simulink model "hcc_sm_v6_circuit"  (R2024b)
settings: Solver=VariableStepAuto  StartTime=0.0  StopTime=1  RelTol=1e-3
libraries: spsSeriesRLCBranchLib x530, spsGtoLib x144, spsNonlinearResistorLib x78, spsGroundLib x2, spsDCVoltageSourceLib x1, spsThreePhaseTransformerTwoWindingsLib x1, spsThreePhaseSourceLib x1, spspowerguiLib x1
(part 1 of 3)
settings Model: Creator=56305  LastModifiedBy=XixiLab
settings OptimizationCC: ReuseModelBlockBuffer=off
settings RTWCC: GPUComputeCapability=3.5

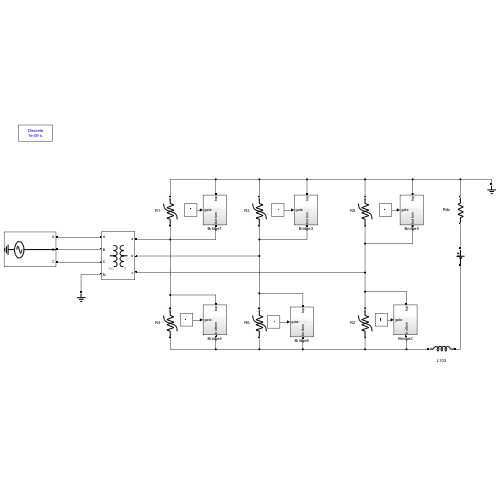
[thumbnail: Simulink's stored preview of the top-level diagram]
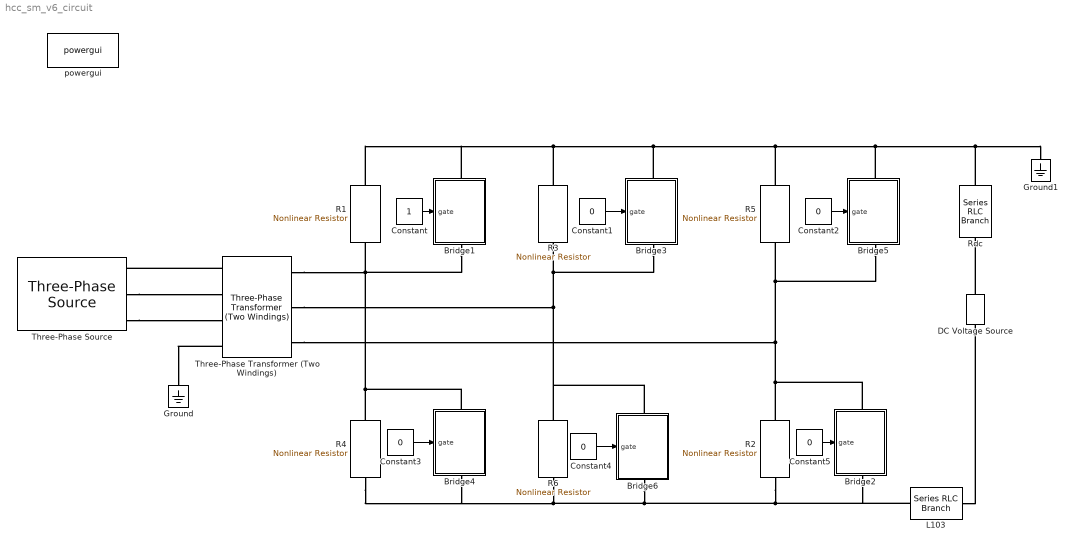
== system hcc_sm_v6_circuit ==
  Bridge1 : Subsystem
      settings: PortSchema="{\"entries\":[{\"content\":{\"sides\":[{\"content\":{\"connectorIds\":[\"In1\"]},\"type\":\"ConnectorPlacement.EquallySpacedRectSide\",\"uuid\":\"41aa3e2a-70f0-4b77-aa16-68e99ec54bcf\"},{\"content\":{\"side\":\"RIGHT\"},\"type\":\"ConnectorPlacement.EquallySpacedRectSide\",\"uuid\":\"96eb3ac2-20ab-4313-b955-709dae12ba5a\"},{\"content\":{\"connectorIds\":[\"LConn1\"],\"side\":\"TOP\"},\"type\":\"ConnectorPlacement.EquallySpacedRectSide\",\"uuid\":\"75cf1ed1-d1d6-43fb-a0f7-eae0627f950f\"},{\"content\":{\"connectorIds\":[\"RConn1\"],\"side\":\"BOTTOM\"},\"type\":\"ConnectorPlacement.EquallySpacedRectSide\",\"uuid\":\"e3d24c16-695e-4958-a9e5-c1041aebacaf\"}]},\"type\":\"ConnectorPlacement.EquallySpacedConnector\",\"uuid\":\"cea135f8-b684-4f22-bc6f-773380cf8880\"}],\"packageUris\":[\"http://schema.mathworks.com/mf0/Connector/R2020b\"],\"version\":\"1.0\"}"
  Bridge2 : Subsystem
      settings: PortSchema="{\"entries\":[{\"content\":{\"sides\":[{\"content\":{\"connectorIds\":[\"In1\"]},\"type\":\"ConnectorPlacement.EquallySpacedRectSide\",\"uuid\":\"41aa3e2a-70f0-4b77-aa16-68e99ec54bcf\"},{\"content\":{\"side\":\"RIGHT\"},\"type\":\"ConnectorPlacement.EquallySpacedRectSide\",\"uuid\":\"96eb3ac2-20ab-4313-b955-709dae12ba5a\"},{\"content\":{\"connectorIds\":[\"LConn1\"],\"side\":\"TOP\"},\"type\":\"ConnectorPlacement.EquallySpacedRectSide\",\"uuid\":\"75cf1ed1-d1d6-43fb-a0f7-eae0627f950f\"},{\"content\":{\"connectorIds\":[\"RConn1\"],\"side\":\"BOTTOM\"},\"type\":\"ConnectorPlacement.EquallySpacedRectSide\",\"uuid\":\"e3d24c16-695e-4958-a9e5-c1041aebacaf\"}]},\"type\":\"ConnectorPlacement.EquallySpacedConnector\",\"uuid\":\"cea135f8-b684-4f22-bc6f-773380cf8880\"}],\"packageUris\":[\"http://schema.mathworks.com/mf0/Connector/R2020b\"],\"version\":\"1.0\"}"
  Bridge3 : Subsystem
      settings: PortSchema="{\"entries\":[{\"content\":{\"sides\":[{\"content\":{\"connectorIds\":[\"In1\"]},\"type\":\"ConnectorPlacement.EquallySpacedRectSide\",\"uuid\":\"41aa3e2a-70f0-4b77-aa16-68e99ec54bcf\"},{\"content\":{\"side\":\"RIGHT\"},\"type\":\"ConnectorPlacement.EquallySpacedRectSide\",\"uuid\":\"96eb3ac2-20ab-4313-b955-709dae12ba5a\"},{\"content\":{\"connectorIds\":[\"LConn1\"],\"side\":\"TOP\"},\"type\":\"ConnectorPlacement.EquallySpacedRectSide\",\"uuid\":\"75cf1ed1-d1d6-43fb-a0f7-eae0627f950f\"},{\"content\":{\"connectorIds\":[\"RConn1\"],\"side\":\"BOTTOM\"},\"type\":\"ConnectorPlacement.EquallySpacedRectSide\",\"uuid\":\"e3d24c16-695e-4958-a9e5-c1041aebacaf\"}]},\"type\":\"ConnectorPlacement.EquallySpacedConnector\",\"uuid\":\"cea135f8-b684-4f22-bc6f-773380cf8880\"}],\"packageUris\":[\"http://schema.mathworks.com/mf0/Connector/R2020b\"],\"version\":\"1.0\"}"
  Bridge4 : Subsystem
      settings: PortSchema="{\"entries\":[{\"content\":{\"sides\":[{\"content\":{\"connectorIds\":[\"In1\"]},\"type\":\"ConnectorPlacement.EquallySpacedRectSide\",\"uuid\":\"41aa3e2a-70f0-4b77-aa16-68e99ec54bcf\"},{\"content\":{\"side\":\"RIGHT\"},\"type\":\"ConnectorPlacement.EquallySpacedRectSide\",\"uuid\":\"96eb3ac2-20ab-4313-b955-709dae12ba5a\"},{\"content\":{\"connectorIds\":[\"LConn1\"],\"side\":\"TOP\"},\"type\":\"ConnectorPlacement.EquallySpacedRectSide\",\"uuid\":\"75cf1ed1-d1d6-43fb-a0f7-eae0627f950f\"},{\"content\":{\"connectorIds\":[\"RConn1\"],\"side\":\"BOTTOM\"},\"type\":\"ConnectorPlacement.EquallySpacedRectSide\",\"uuid\":\"e3d24c16-695e-4958-a9e5-c1041aebacaf\"}]},\"type\":\"ConnectorPlacement.EquallySpacedConnector\",\"uuid\":\"cea135f8-b684-4f22-bc6f-773380cf8880\"}],\"packageUris\":[\"http://schema.mathworks.com/mf0/Connector/R2020b\"],\"version\":\"1.0\"}"
  Bridge5 : Subsystem
      settings: PortSchema="{\"entries\":[{\"content\":{\"sides\":[{\"content\":{\"connectorIds\":[\"In1\"]},\"type\":\"ConnectorPlacement.EquallySpacedRectSide\",\"uuid\":\"41aa3e2a-70f0-4b77-aa16-68e99ec54bcf\"},{\"content\":{\"side\":\"RIGHT\"},\"type\":\"ConnectorPlacement.EquallySpacedRectSide\",\"uuid\":\"96eb3ac2-20ab-4313-b955-709dae12ba5a\"},{\"content\":{\"connectorIds\":[\"LConn1\"],\"side\":\"TOP\"},\"type\":\"ConnectorPlacement.EquallySpacedRectSide\",\"uuid\":\"75cf1ed1-d1d6-43fb-a0f7-eae0627f950f\"},{\"content\":{\"connectorIds\":[\"RConn1\"],\"side\":\"BOTTOM\"},\"type\":\"ConnectorPlacement.EquallySpacedRectSide\",\"uuid\":\"e3d24c16-695e-4958-a9e5-c1041aebacaf\"}]},\"type\":\"ConnectorPlacement.EquallySpacedConnector\",\"uuid\":\"cea135f8-b684-4f22-bc6f-773380cf8880\"}],\"packageUris\":[\"http://schema.mathworks.com/mf0/Connector/R2020b\"],\"version\":\"1.0\"}"
  Bridge6 : Subsystem
      settings: PortSchema="{\"entries\":[{\"content\":{\"sides\":[{\"content\":{\"connectorIds\":[\"In1\"]},\"type\":\"ConnectorPlacement.EquallySpacedRectSide\",\"uuid\":\"41aa3e2a-70f0-4b77-aa16-68e99ec54bcf\"},{\"content\":{\"side\":\"RIGHT\"},\"type\":\"ConnectorPlacement.EquallySpacedRectSide\",\"uuid\":\"96eb3ac2-20ab-4313-b955-709dae12ba5a\"},{\"content\":{\"connectorIds\":[\"LConn1\"],\"side\":\"TOP\"},\"type\":\"ConnectorPlacement.EquallySpacedRectSide\",\"uuid\":\"75cf1ed1-d1d6-43fb-a0f7-eae0627f950f\"},{\"content\":{\"connectorIds\":[\"RConn1\"],\"side\":\"BOTTOM\"},\"type\":\"ConnectorPlacement.EquallySpacedRectSide\",\"uuid\":\"e3d24c16-695e-4958-a9e5-c1041aebacaf\"}]},\"type\":\"ConnectorPlacement.EquallySpacedConnector\",\"uuid\":\"cea135f8-b684-4f22-bc6f-773380cf8880\"}],\"packageUris\":[\"http://schema.mathworks.com/mf0/Connector/R2020b\"],\"version\":\"1.0\"}"
  Constant : Constant
  Constant{1..5} (5 alike) : Constant  Value=0
  DC Voltage Source : spsDCVoltageSourceLib/DC Voltage Source  Amplitude=5700  Measurements=None
  Ground : spsGroundLib/Ground  LConnTagsString=a
  Ground1 : spsGroundLib/Ground  LConnTagsString=a
  L103 : spsSeriesRLCBranchLib/Series RLC Branch  LConnTagsString=__new0  RConnTagsString=__new0  BranchType=L  Resistance=36  Inductance=120e-03  SetiL0=off  InitialCurrent=0  Capacitance=2.62e-06  Setx0=off  InitialVoltage=0  Measurements=None
  R{1..6} (6 alike) : spsNonlinearResistorLib/Nonlinear Resistor  SrcType=Current source  VI=[9800 0.001;11564 200;12299 1000;13259.4098 4000.01;13259.4196 4000.02;13259.4294 4000.03;13259.4392 4000.04;13259.449 4000.05;13259.4588 4000.06;13259.4686 4000.07;13259.4784 4000.08]
      settings: LibrarySourceBlock=sps_lib/Passives/Nonlinear Resistor
  Rdc : spsSeriesRLCBranchLib/Series RLC Branch  LConnTagsString=__new0  RConnTagsString=__new0  BranchType=R  Resistance=1  Inductance=120e-03  SetiL0=off  InitialCurrent=0  Capacitance=2.62e-06  Setx0=off  InitialVoltage=0  Measurements=None
  Three-Phase Transformer (Two Windings) : spsThreePhaseTransformerTwoWindingsLib/Three-Phase Transformer (Two Windings)  Winding1Connection=Yn  Winding2Connection=Y  CoreType=Three single-phase transformers  SetSaturation=off  Hysteresis=off  DataFile='hysteresis'  SetInitialFlux=off  Measurements=None  UNITS=pu  NominalPower=[ 215.4e6 , 50 ]  Winding1=[ 345e3 , 0.002 , 0.08 ]  Winding2=[ 50.8e3 , 0.002 , 0.08 ]  Rm=500  Lm=500  L0=0.5  Saturation=[ 0,0 ; 0.0024,1.2 ; 1.0,1.52 ]  InitialFluxes=[ 0.8 , -0.8 , 0.7 ]  BreakLoop=off  DiscreteSolver=Trapezoidal iterative  DataType=off  TransfoNumber=1
  Three-Phase Source : spsThreePhaseSourceLib/Three-Phase Source  InternalConnection=Yg  VoltagePhases=off  Voltage=345e3  PhaseAngle=0  Voltage_phases=[25e3 25e3 25e3]/sqrt(3)  PhaseAngles_phases=[0 -120 +120]  Frequency=50  NonIdealSource=off  SpecifyImpedance=off  Resistance=0  Inductance=0  ShortCircuitLevel=100e6  BaseVoltage=25e3  XRratio=7  BusType=swing  Pref=10e3  Qref=0  Prefabc=[10e3, 10e3, 10e3]  Qrefabc=[0, 0, 0]  Qmin=-inf  Qmax=inf
  powergui : spspowerguiLib/powergui  Priority=1  SimulationMode=Discrete  SampleTime=1e-9  frequency=60  Iterations=50  frequencyindice=0  Pbase=100e6  ErrMax=1e-4  UnitsV=kV  UnitsW=MW  buscounter=0  FunctionMessages=off  echomessages=off  EnableUseOfTLC=off  CurrentSourceSwitches=off  DisableSnubberDevices=off  DisableRonSwitches=off  DisableVfSwitches=off  DisplayEquations=off  AutomaticDiscreteSolvers=off  SolverType=Tustin/Backward Euler (TBE)  Interpol=off  ExternalGateDelay=off  methode=off  Ts=100  x0status=blocks  SPID=on  SwTol=0  HookPort=off  NonlinearTolerance=1e-4  nMaxIteration=100  ContinueOnMaxIteration=off  RestoreLinks=warning  ResistiveCurrentMeasurement=off  Frange=[0:2:500]  Ylog=off  Xlog=on  ShowGrid=off  save=off  variable=ZData  structure=0  ZoomFFT=off  StartTime=0.0  cycles=1  DisplayStyle=1  fundamental=60  FreqAxis=off  MaxFrequency=1000  frequencyindicesteady=1  RmsSteady=1  display=off
  wires:
  Constant/1 -> Bridge1/1(gate)
  Constant1/1 -> Bridge3/1(gate)
  Constant2/1 -> Bridge5/1(gate)
  Constant3/1 -> Bridge4/1(gate)
  Constant4/1 -> Bridge6/1(gate)
  Constant5/1 -> Bridge2/1(gate)
  connections:
  Three-Phase Transformer (Two Windings)/LConn1 -- Three-Phase Source/RConn1
  Three-Phase Source/RConn2 -- Three-Phase Transformer (Two Windings)/LConn2
  Three-Phase Source/RConn3 -- Three-Phase Transformer (Two Windings)/LConn3
  Three-Phase Transformer (Two Windings)/LConn4 -- Ground/LConn1
  R4/LConn1 -- Bridge4/LConn1 -- Bridge1/RConn1 -- R1/RConn1 -- Three-Phase Transformer (Two Windings)/RConn1
  Three-Phase Transformer (Two Windings)/RConn2 -- Bridge6/LConn1 -- R6/LConn1 -- Bridge3/RConn1 -- R3/RConn1
  R2/LConn1 -- Bridge2/LConn1 -- Three-Phase Transformer (Two Windings)/RConn3 -- Bridge5/RConn1 -- R5/RConn1
  R2/RConn1 -- Bridge2/RConn1 -- L103/LConn1 -- Bridge6/RConn1 -- Bridge4/RConn1 -- R4/RConn1 -- R6/RConn1
  DC Voltage Source/RConn1 -- Rdc/RConn1
  R3/LConn1 -- R1/LConn1 -- Bridge1/LConn1 -- Bridge3/LConn1 -- R5/LConn1 -- Bridge5/LConn1 -- Rdc/LConn1 -- Ground1/LConn1
  L103/RConn1 -- DC Voltage Source/LConn1

== system hcc_sm_v6_circuit/Bridge1 ==
  gate : Inport
  Segment1 : Subsystem
  Segment2 : Subsystem
  Segment3 : Subsystem
  Segment4 : Subsystem
  top : PMIOPort  Side=Left
  bottom : PMIOPort  Port=2  Side=Right
  wires:
  gate/1 -> Segment2/1(gate), Segment4/1(gate), Segment3/1(gate), Segment1/1(gate)
  connections:
  Segment2/LConn1 -- Segment1/RConn1
  Segment3/LConn1 -- Segment2/RConn1
  Segment4/LConn1 -- Segment3/RConn1
  top/RConn1 -- Segment1/LConn1
  Segment4/RConn1 -- bottom/RConn1

== system hcc_sm_v6_circuit/Bridge2 ==
  gate : Inport
  Segment1 : Subsystem
  Segment2 : Subsystem
  Segment3 : Subsystem
  Segment4 : Subsystem
  top : PMIOPort  Side=Left
  bottom : PMIOPort  Port=2  Side=Right
  wires:
  gate/1 -> Segment2/1(gate), Segment4/1(gate), Segment3/1(gate), Segment1/1(gate)
  connections:
  Segment2/LConn1 -- Segment1/RConn1
  Segment3/LConn1 -- Segment2/RConn1
  Segment4/LConn1 -- Segment3/RConn1
  top/RConn1 -- Segment1/LConn1
  Segment4/RConn1 -- bottom/RConn1

== system hcc_sm_v6_circuit/Bridge3 ==
  gate : Inport
  Segment1 : Subsystem
  Segment2 : Subsystem
  Segment3 : Subsystem
  Segment4 : Subsystem
  top : PMIOPort  Side=Left
  bottom : PMIOPort  Port=2  Side=Right
  wires:
  gate/1 -> Segment2/1(gate), Segment4/1(gate), Segment3/1(gate), Segment1/1(gate)
  connections:
  Segment2/LConn1 -- Segment1/RConn1
  Segment3/LConn1 -- Segment2/RConn1
  Segment4/LConn1 -- Segment3/RConn1
  top/RConn1 -- Segment1/LConn1
  Segment4/RConn1 -- bottom/RConn1

== system hcc_sm_v6_circuit/Bridge4 ==
  gate : Inport
  Segment1 : Subsystem
  Segment2 : Subsystem
  Segment3 : Subsystem
  Segment4 : Subsystem
  top : PMIOPort  Side=Left
  bottom : PMIOPort  Port=2  Side=Right
  wires:
  gate/1 -> Segment2/1(gate), Segment4/1(gate), Segment3/1(gate), Segment1/1(gate)
  connections:
  Segment2/LConn1 -- Segment1/RConn1
  Segment3/LConn1 -- Segment2/RConn1
  Segment4/LConn1 -- Segment3/RConn1
  top/RConn1 -- Segment1/LConn1
  Segment4/RConn1 -- bottom/RConn1

== system hcc_sm_v6_circuit/Bridge5 ==
  gate : Inport
  Segment1 : Subsystem
  Segment2 : Subsystem
  Segment3 : Subsystem
  Segment4 : Subsystem
  top : PMIOPort  Side=Left
  bottom : PMIOPort  Port=2  Side=Right
  wires:
  gate/1 -> Segment2/1(gate), Segment4/1(gate), Segment3/1(gate), Segment1/1(gate)
  connections:
  Segment2/LConn1 -- Segment1/RConn1
  Segment3/LConn1 -- Segment2/RConn1
  Segment4/LConn1 -- Segment3/RConn1
  top/RConn1 -- Segment1/LConn1
  Segment4/RConn1 -- bottom/RConn1

== system hcc_sm_v6_circuit/Bridge6 ==
  gate : Inport
  Segment1 : Subsystem
  Segment2 : Subsystem
  Segment3 : Subsystem
  Segment4 : Subsystem
  top : PMIOPort  Side=Left
  bottom : PMIOPort  Port=2  Side=Right
  wires:
  gate/1 -> Segment2/1(gate), Segment4/1(gate), Segment3/1(gate), Segment1/1(gate)
  connections:
  Segment2/LConn1 -- Segment1/RConn1
  Segment3/LConn1 -- Segment2/RConn1
  Segment4/LConn1 -- Segment3/RConn1
  top/RConn1 -- Segment1/LConn1
  Segment4/RConn1 -- bottom/RConn1

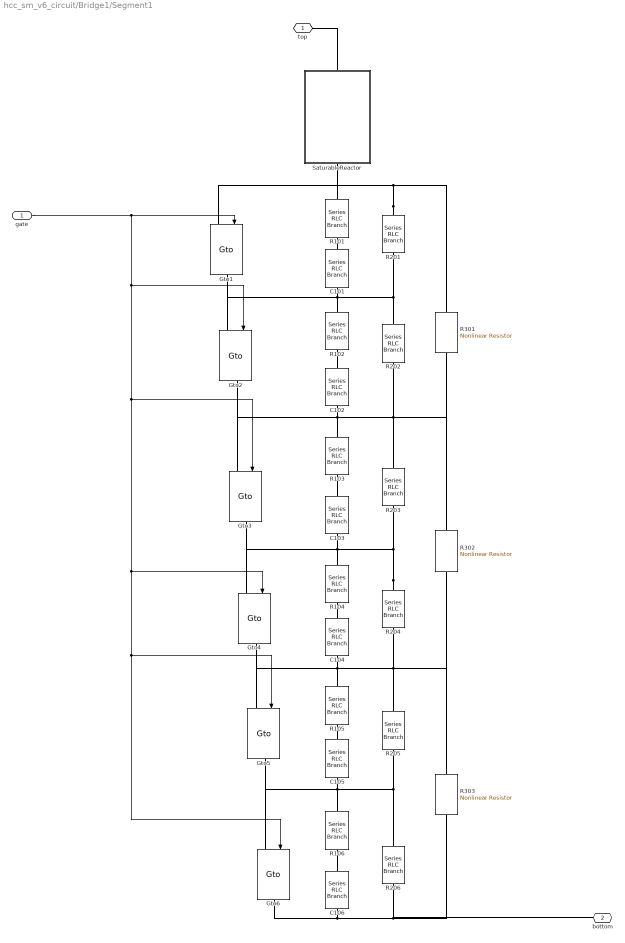
== system hcc_sm_v6_circuit/Bridge1/Segment1 ==
  gate : Inport
  C{101..106} (6 alike) : spsSeriesRLCBranchLib/Series RLC Branch  LConnTagsString=__new0  RConnTagsString=__new0  BranchType=C  Resistance=350  Inductance=107.42e-03  SetiL0=off  InitialCurrent=0  Capacitance=2.2*1e-6  Setx0=off  InitialVoltage=0  Measurements=None
  Gto{1..6} (6 alike) : spsGtoLib/Gto  Ron=0.226e-6  Lon=0  Vf=1.2  Tf=10e-6  Tt=20e-6  IC=0  Rs=161.25e3  Cs=0  Measurements=off
      settings: LibrarySourceBlock=sps_lib/Power Electronics/Gto
  R{101..106} (6 alike) : spsSeriesRLCBranchLib/Series RLC Branch  LConnTagsString=__new0  RConnTagsString=__new0  BranchType=R  Resistance=36  Inductance=107.42e-03  SetiL0=off  InitialCurrent=0  Capacitance=2.62e-06  Setx0=off  InitialVoltage=0  Measurements=None
  R{201..206} (6 alike) : spsSeriesRLCBranchLib/Series RLC Branch  LConnTagsString=__new0  RConnTagsString=__new0  BranchType=R  Resistance=88  Inductance=107.42e-03  SetiL0=off  InitialCurrent=0  Capacitance=2.62e-06  Setx0=off  InitialVoltage=0  Measurements=None
  R301 : spsNonlinearResistorLib/Nonlinear Resistor  SrcType=Current source  VI=[4400 0.001;5199.92 10;5449.84 100;5700.2 250;5849.8 500;5925.04 750;5999.84 1000;6199.64 2000;6274.84 2500;6325 3000;6600 5500]
      settings: LibrarySourceBlock=sps_lib/Passives/Nonlinear Resistor
  R302 : spsNonlinearResistorLib/Nonlinear Resistor  SrcType=Current source  VI=[4400 0.001;5199.92 10;5449.84 100;5700.2 250;5849.8 500;5925.04 750;5999.84 1000;6199.64 2000;6274.84 2500;6325 3000;6600 5500]
      settings: LibrarySourceBlock=sps_lib/Passives/Nonlinear Resistor
  R303 : spsNonlinearResistorLib/Nonlinear Resistor  SrcType=Current source  VI=[4400 0.001;5199.92 10;5449.84 100;5700.2 250;5849.8 500;5925.04 750;5999.84 1000;6199.64 2000;6274.84 2500;6325 3000;6600 5500]
      settings: LibrarySourceBlock=sps_lib/Passives/Nonlinear Resistor
  SaturableReactor : Subsystem
  top : PMIOPort  Side=Left
  bottom : PMIOPort  Port=2  Side=Right
  wires:
  gate/1 -> Gto3/1, Gto4/1, Gto6/1, Gto5/1, Gto2/1, Gto1/1
  connections:
  R201/RConn1 -- Gto2/LConn1 -- Gto1/RConn1 -- C101/RConn1 -- R102/LConn1 -- R202/LConn1
  R204/LConn1 -- R203/RConn1 -- C103/RConn1 -- Gto4/LConn1 -- Gto3/RConn1 -- R104/LConn1
  R201/LConn1 -- R301/LConn1 -- Gto1/LConn1 -- SaturableReactor/RConn1 -- R101/LConn1
  R205/RConn1 -- C105/RConn1 -- R106/LConn1 -- Gto6/LConn1 -- Gto5/RConn1 -- R206/LConn1
  R202/RConn1 -- R203/LConn1 -- R302/LConn1 -- R301/RConn1 -- C102/RConn1 -- Gto3/LConn1 -- Gto2/RConn1 -- R103/LConn1
  R105/LConn1 -- C104/RConn1 -- Gto5/LConn1 -- Gto4/RConn1 -- R205/LConn1 -- R303/LConn1 -- R302/RConn1 -- R204/RConn1
  R303/RConn1 -- bottom/RConn1 -- R206/RConn1 -- C106/RConn1 -- Gto6/RConn1
  SaturableReactor/LConn1 -- top/RConn1
  C101/LConn1 -- R101/RConn1
  C102/LConn1 -- R102/RConn1
  R103/RConn1 -- C103/LConn1
  R104/RConn1 -- C104/LConn1
  R105/RConn1 -- C105/LConn1
  R106/RConn1 -- C106/LConn1

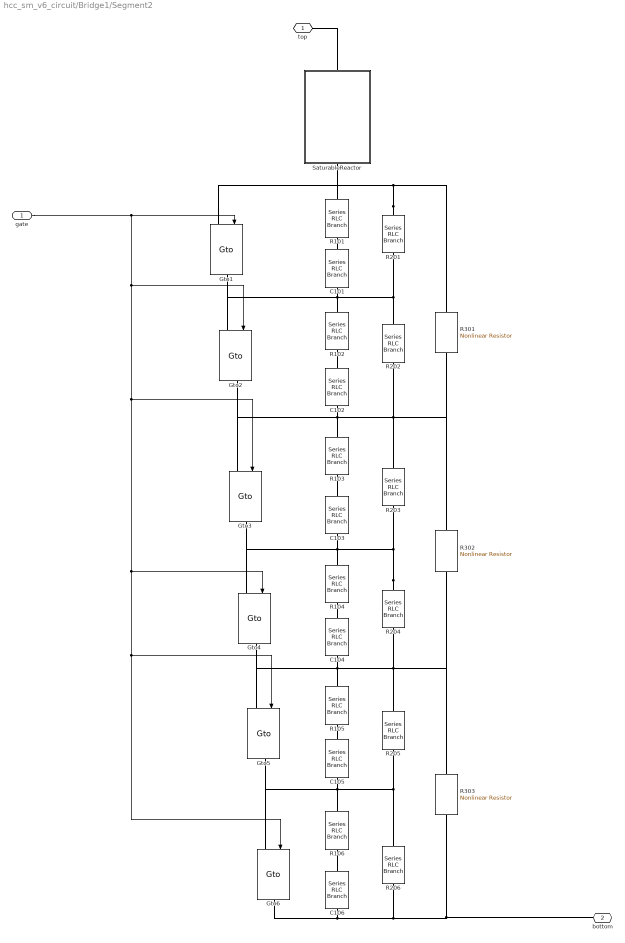
== system hcc_sm_v6_circuit/Bridge1/Segment2 ==
  gate : Inport
  C{101..106} (6 alike) : spsSeriesRLCBranchLib/Series RLC Branch  LConnTagsString=__new0  RConnTagsString=__new0  BranchType=C  Resistance=350  Inductance=107.42e-03  SetiL0=off  InitialCurrent=0  Capacitance=2.2*1e-6  Setx0=off  InitialVoltage=0  Measurements=None
  Gto{1..6} (6 alike) : spsGtoLib/Gto  Ron=0.226e-6  Lon=0  Vf=1.2  Tf=10e-6  Tt=20e-6  IC=0  Rs=161.25e3  Cs=0  Measurements=off
  R{101..106} (6 alike) : spsSeriesRLCBranchLib/Series RLC Branch  LConnTagsString=__new0  RConnTagsString=__new0  BranchType=R  Resistance=36  Inductance=107.42e-03  SetiL0=off  InitialCurrent=0  Capacitance=2.62e-06  Setx0=off  InitialVoltage=0  Measurements=None
  R{201..206} (6 alike) : spsSeriesRLCBranchLib/Series RLC Branch  LConnTagsString=__new0  RConnTagsString=__new0  BranchType=R  Resistance=88  Inductance=107.42e-03  SetiL0=off  InitialCurrent=0  Capacitance=2.62e-06  Setx0=off  InitialVoltage=0  Measurements=None
  R301 : spsNonlinearResistorLib/Nonlinear Resistor  SrcType=Current source  VI=[4400 0.001;5199.92 10;5449.84 100;5700.2 250;5849.8 500;5925.04 750;5999.84 1000;6199.64 2000;6274.84 2500;6325 3000;6600 5500]
  R302 : spsNonlinearResistorLib/Nonlinear Resistor  SrcType=Current source  VI=[4400 0.001;5199.92 10;5449.84 100;5700.2 250;5849.8 500;5925.04 750;5999.84 1000;6199.64 2000;6274.84 2500;6325 3000;6600 5500]
  R303 : spsNonlinearResistorLib/Nonlinear Resistor  SrcType=Current source  VI=[4400 0.001;5199.92 10;5449.84 100;5700.2 250;5849.8 500;5925.04 750;5999.84 1000;6199.64 2000;6274.84 2500;6325 3000;6600 5500]
  SaturableReactor : Subsystem
  top : PMIOPort  Side=Left
  bottom : PMIOPort  Port=2  Side=Right
  wires:
  gate/1 -> Gto3/1, Gto4/1, Gto6/1, Gto5/1, Gto2/1, Gto1/1
  connections:
  R201/RConn1 -- Gto2/LConn1 -- Gto1/RConn1 -- C101/RConn1 -- R102/LConn1 -- R202/LConn1
  R204/LConn1 -- R203/RConn1 -- C103/RConn1 -- Gto4/LConn1 -- Gto3/RConn1 -- R104/LConn1
  R201/LConn1 -- R301/LConn1 -- Gto1/LConn1 -- SaturableReactor/RConn1 -- R101/LConn1
  R205/RConn1 -- C105/RConn1 -- R106/LConn1 -- Gto6/LConn1 -- Gto5/RConn1 -- R206/LConn1
  R202/RConn1 -- R203/LConn1 -- R302/LConn1 -- R301/RConn1 -- C102/RConn1 -- Gto3/LConn1 -- Gto2/RConn1 -- R103/LConn1
  R105/LConn1 -- C104/RConn1 -- Gto5/LConn1 -- Gto4/RConn1 -- R205/LConn1 -- R303/LConn1 -- R302/RConn1 -- R204/RConn1
  R303/RConn1 -- bottom/RConn1 -- R206/RConn1 -- C106/RConn1 -- Gto6/RConn1
  SaturableReactor/LConn1 -- top/RConn1
  C101/LConn1 -- R101/RConn1
  C102/LConn1 -- R102/RConn1
  R103/RConn1 -- C103/LConn1
  R104/RConn1 -- C104/LConn1
  R105/RConn1 -- C105/LConn1
  R106/RConn1 -- C106/LConn1

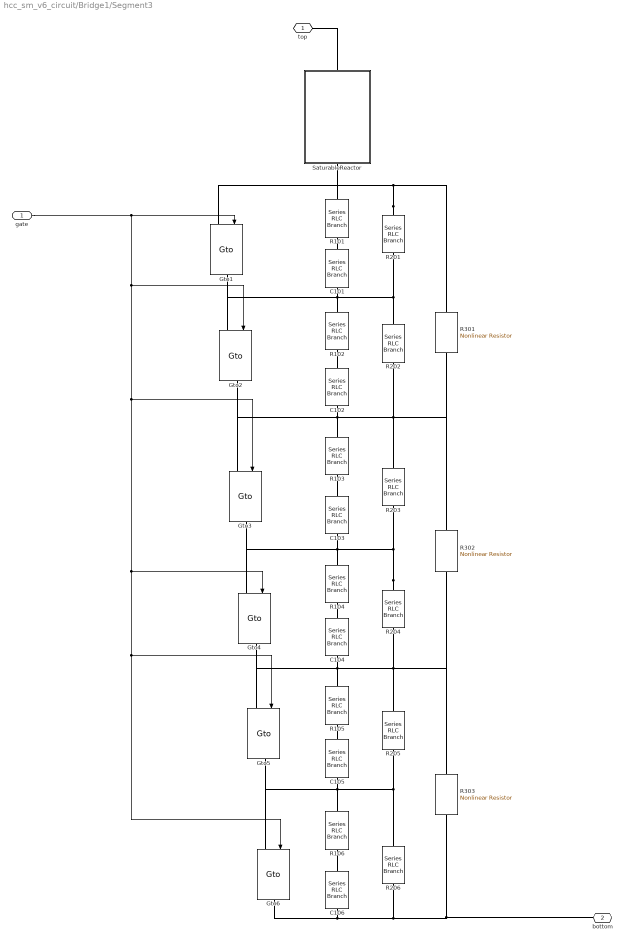
== system hcc_sm_v6_circuit/Bridge1/Segment3 ==
  gate : Inport
  C{101..106} (6 alike) : spsSeriesRLCBranchLib/Series RLC Branch  LConnTagsString=__new0  RConnTagsString=__new0  BranchType=C  Resistance=350  Inductance=107.42e-03  SetiL0=off  InitialCurrent=0  Capacitance=2.2*1e-6  Setx0=off  InitialVoltage=0  Measurements=None
  Gto{1..6} (6 alike) : spsGtoLib/Gto  Ron=0.226e-6  Lon=0  Vf=1.2  Tf=10e-6  Tt=20e-6  IC=0  Rs=161.25e3  Cs=0  Measurements=off
  R{101..106} (6 alike) : spsSeriesRLCBranchLib/Series RLC Branch  LConnTagsString=__new0  RConnTagsString=__new0  BranchType=R  Resistance=36  Inductance=107.42e-03  SetiL0=off  InitialCurrent=0  Capacitance=2.62e-06  Setx0=off  InitialVoltage=0  Measurements=None
  R{201..206} (6 alike) : spsSeriesRLCBranchLib/Series RLC Branch  LConnTagsString=__new0  RConnTagsString=__new0  BranchType=R  Resistance=88  Inductance=107.42e-03  SetiL0=off  InitialCurrent=0  Capacitance=2.62e-06  Setx0=off  InitialVoltage=0  Measurements=None
  R301 : spsNonlinearResistorLib/Nonlinear Resistor  SrcType=Current source  VI=[4400 0.001;5199.92 10;5449.84 100;5700.2 250;5849.8 500;5925.04 750;5999.84 1000;6199.64 2000;6274.84 2500;6325 3000;6600 5500]
  R302 : spsNonlinearResistorLib/Nonlinear Resistor  SrcType=Current source  VI=[4400 0.001;5199.92 10;5449.84 100;5700.2 250;5849.8 500;5925.04 750;5999.84 1000;6199.64 2000;6274.84 2500;6325 3000;6600 5500]
  R303 : spsNonlinearResistorLib/Nonlinear Resistor  SrcType=Current source  VI=[4400 0.001;5199.92 10;5449.84 100;5700.2 250;5849.8 500;5925.04 750;5999.84 1000;6199.64 2000;6274.84 2500;6325 3000;6600 5500]
  SaturableReactor : Subsystem
  top : PMIOPort  Side=Left
  bottom : PMIOPort  Port=2  Side=Right
  wires:
  gate/1 -> Gto3/1, Gto4/1, Gto6/1, Gto5/1, Gto2/1, Gto1/1
  connections:
  R201/RConn1 -- Gto2/LConn1 -- Gto1/RConn1 -- C101/RConn1 -- R102/LConn1 -- R202/LConn1
  R204/LConn1 -- R203/RConn1 -- C103/RConn1 -- Gto4/LConn1 -- Gto3/RConn1 -- R104/LConn1
  R201/LConn1 -- R301/LConn1 -- Gto1/LConn1 -- SaturableReactor/RConn1 -- R101/LConn1
  R205/RConn1 -- C105/RConn1 -- R106/LConn1 -- Gto6/LConn1 -- Gto5/RConn1 -- R206/LConn1
  R202/RConn1 -- R203/LConn1 -- R302/LConn1 -- R301/RConn1 -- C102/RConn1 -- Gto3/LConn1 -- Gto2/RConn1 -- R103/LConn1
  R105/LConn1 -- C104/RConn1 -- Gto5/LConn1 -- Gto4/RConn1 -- R205/LConn1 -- R303/LConn1 -- R302/RConn1 -- R204/RConn1
  R303/RConn1 -- bottom/RConn1 -- R206/RConn1 -- C106/RConn1 -- Gto6/RConn1
  SaturableReactor/LConn1 -- top/RConn1
  C101/LConn1 -- R101/RConn1
  C102/LConn1 -- R102/RConn1
  R103/RConn1 -- C103/LConn1
  R104/RConn1 -- C104/LConn1
  R105/RConn1 -- C105/LConn1
  R106/RConn1 -- C106/LConn1

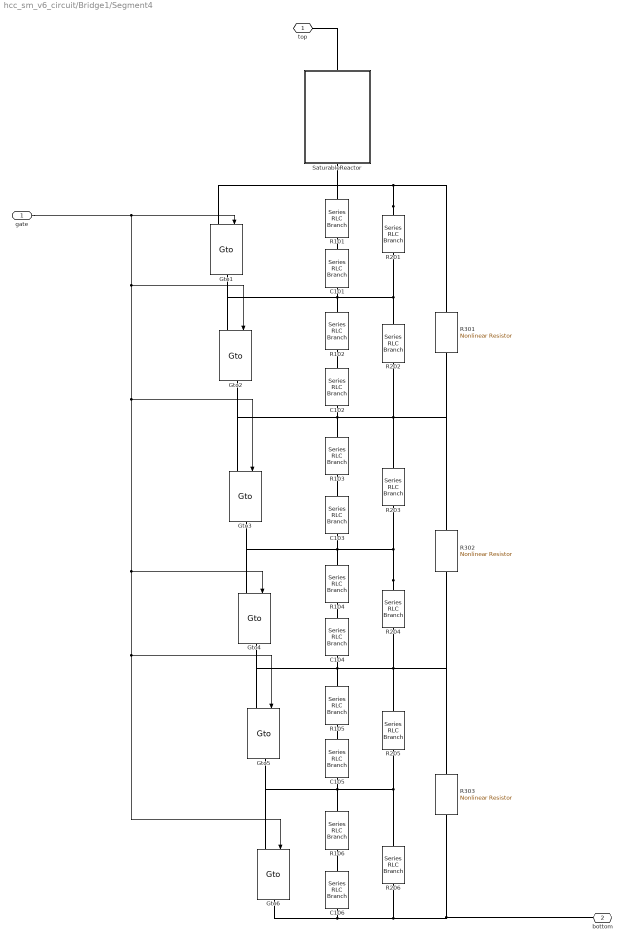
== system hcc_sm_v6_circuit/Bridge1/Segment4 ==
  gate : Inport
  C{101..106} (6 alike) : spsSeriesRLCBranchLib/Series RLC Branch  LConnTagsString=__new0  RConnTagsString=__new0  BranchType=C  Resistance=350  Inductance=107.42e-03  SetiL0=off  InitialCurrent=0  Capacitance=2.2*1e-6  Setx0=off  InitialVoltage=0  Measurements=None
  Gto{1..6} (6 alike) : spsGtoLib/Gto  Ron=0.226e-6  Lon=0  Vf=1.2  Tf=10e-6  Tt=20e-6  IC=0  Rs=161.25e3  Cs=0  Measurements=off
  R{101..106} (6 alike) : spsSeriesRLCBranchLib/Series RLC Branch  LConnTagsString=__new0  RConnTagsString=__new0  BranchType=R  Resistance=36  Inductance=107.42e-03  SetiL0=off  InitialCurrent=0  Capacitance=2.62e-06  Setx0=off  InitialVoltage=0  Measurements=None
  R{201..206} (6 alike) : spsSeriesRLCBranchLib/Series RLC Branch  LConnTagsString=__new0  RConnTagsString=__new0  BranchType=R  Resistance=88  Inductance=107.42e-03  SetiL0=off  InitialCurrent=0  Capacitance=2.62e-06  Setx0=off  InitialVoltage=0  Measurements=None
  R301 : spsNonlinearResistorLib/Nonlinear Resistor  SrcType=Current source  VI=[4400 0.001;5199.92 10;5449.84 100;5700.2 250;5849.8 500;5925.04 750;5999.84 1000;6199.64 2000;6274.84 2500;6325 3000;6600 5500]
  R302 : spsNonlinearResistorLib/Nonlinear Resistor  SrcType=Current source  VI=[4400 0.001;5199.92 10;5449.84 100;5700.2 250;5849.8 500;5925.04 750;5999.84 1000;6199.64 2000;6274.84 2500;6325 3000;6600 5500]
  R303 : spsNonlinearResistorLib/Nonlinear Resistor  SrcType=Current source  VI=[4400 0.001;5199.92 10;5449.84 100;5700.2 250;5849.8 500;5925.04 750;5999.84 1000;6199.64 2000;6274.84 2500;6325 3000;6600 5500]
  SaturableReactor : Subsystem
  top : PMIOPort  Side=Left
  bottom : PMIOPort  Port=2  Side=Right
  wires:
  gate/1 -> Gto3/1, Gto4/1, Gto6/1, Gto5/1, Gto2/1, Gto1/1
  connections:
  R201/RConn1 -- Gto2/LConn1 -- Gto1/RConn1 -- C101/RConn1 -- R102/LConn1 -- R202/LConn1
  R204/LConn1 -- R203/RConn1 -- C103/RConn1 -- Gto4/LConn1 -- Gto3/RConn1 -- R104/LConn1
  R201/LConn1 -- R301/LConn1 -- Gto1/LConn1 -- SaturableReactor/RConn1 -- R101/LConn1
  R205/RConn1 -- C105/RConn1 -- R106/LConn1 -- Gto6/LConn1 -- Gto5/RConn1 -- R206/LConn1
  R202/RConn1 -- R203/LConn1 -- R302/LConn1 -- R301/RConn1 -- C102/RConn1 -- Gto3/LConn1 -- Gto2/RConn1 -- R103/LConn1
  R105/LConn1 -- C104/RConn1 -- Gto5/LConn1 -- Gto4/RConn1 -- R205/LConn1 -- R303/LConn1 -- R302/RConn1 -- R204/RConn1
  R303/RConn1 -- bottom/RConn1 -- R206/RConn1 -- C106/RConn1 -- Gto6/RConn1
  SaturableReactor/LConn1 -- top/RConn1
  C101/LConn1 -- R101/RConn1
  C102/LConn1 -- R102/RConn1
  R103/RConn1 -- C103/LConn1
  R104/RConn1 -- C104/LConn1
  R105/RConn1 -- C105/LConn1
  R106/RConn1 -- C106/LConn1

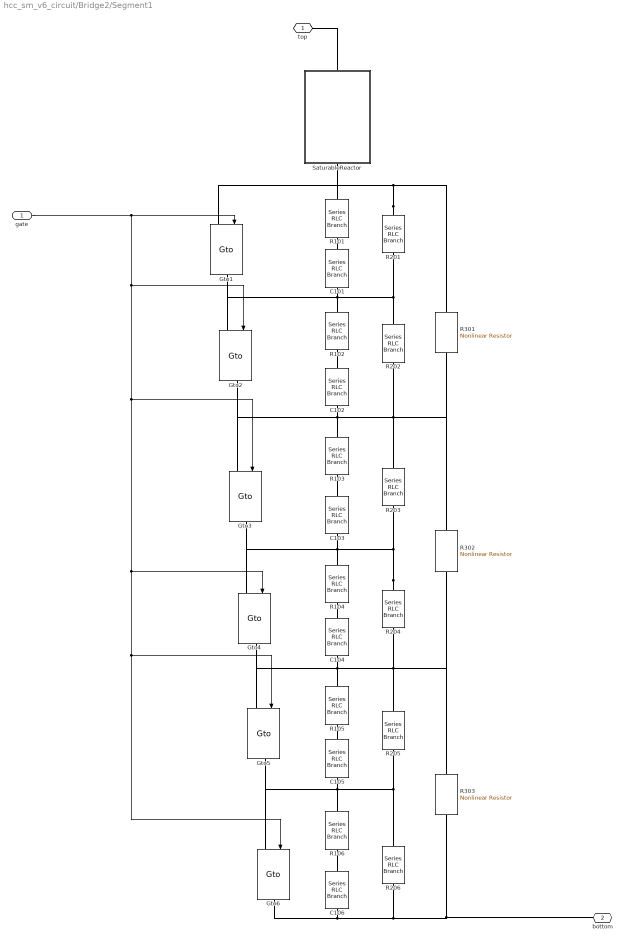
== system hcc_sm_v6_circuit/Bridge2/Segment1 ==
  gate : Inport
  C{101..106} (6 alike) : spsSeriesRLCBranchLib/Series RLC Branch  LConnTagsString=__new0  RConnTagsString=__new0  BranchType=C  Resistance=350  Inductance=107.42e-03  SetiL0=off  InitialCurrent=0  Capacitance=2.2*1e-6  Setx0=off  InitialVoltage=0  Measurements=None
  Gto{1..6} (6 alike) : spsGtoLib/Gto  Ron=0.226e-6  Lon=0  Vf=1.2  Tf=10e-6  Tt=20e-6  IC=0  Rs=161.25e3  Cs=0  Measurements=off
  R{101..106} (6 alike) : spsSeriesRLCBranchLib/Series RLC Branch  LConnTagsString=__new0  RConnTagsString=__new0  BranchType=R  Resistance=36  Inductance=107.42e-03  SetiL0=off  InitialCurrent=0  Capacitance=2.62e-06  Setx0=off  InitialVoltage=0  Measurements=None
  R{201..206} (6 alike) : spsSeriesRLCBranchLib/Series RLC Branch  LConnTagsString=__new0  RConnTagsString=__new0  BranchType=R  Resistance=88  Inductance=107.42e-03  SetiL0=off  InitialCurrent=0  Capacitance=2.62e-06  Setx0=off  InitialVoltage=0  Measurements=None
  R301 : spsNonlinearResistorLib/Nonlinear Resistor  SrcType=Current source  VI=[4400 0.001;5199.92 10;5449.84 100;5700.2 250;5849.8 500;5925.04 750;5999.84 1000;6199.64 2000;6274.84 2500;6325 3000;6600 5500]
  R302 : spsNonlinearResistorLib/Nonlinear Resistor  SrcType=Current source  VI=[4400 0.001;5199.92 10;5449.84 100;5700.2 250;5849.8 500;5925.04 750;5999.84 1000;6199.64 2000;6274.84 2500;6325 3000;6600 5500]
  R303 : spsNonlinearResistorLib/Nonlinear Resistor  SrcType=Current source  VI=[4400 0.001;5199.92 10;5449.84 100;5700.2 250;5849.8 500;5925.04 750;5999.84 1000;6199.64 2000;6274.84 2500;6325 3000;6600 5500]
  SaturableReactor : Subsystem
  top : PMIOPort  Side=Left
  bottom : PMIOPort  Port=2  Side=Right
  wires:
  gate/1 -> Gto3/1, Gto4/1, Gto6/1, Gto5/1, Gto2/1, Gto1/1
  connections:
  R201/RConn1 -- Gto2/LConn1 -- Gto1/RConn1 -- C101/RConn1 -- R102/LConn1 -- R202/LConn1
  R204/LConn1 -- R203/RConn1 -- C103/RConn1 -- Gto4/LConn1 -- Gto3/RConn1 -- R104/LConn1
  R201/LConn1 -- R301/LConn1 -- Gto1/LConn1 -- SaturableReactor/RConn1 -- R101/LConn1
  R205/RConn1 -- C105/RConn1 -- R106/LConn1 -- Gto6/LConn1 -- Gto5/RConn1 -- R206/LConn1
  R202/RConn1 -- R203/LConn1 -- R302/LConn1 -- R301/RConn1 -- C102/RConn1 -- Gto3/LConn1 -- Gto2/RConn1 -- R103/LConn1
  R105/LConn1 -- C104/RConn1 -- Gto5/LConn1 -- Gto4/RConn1 -- R205/LConn1 -- R303/LConn1 -- R302/RConn1 -- R204/RConn1
  R303/RConn1 -- bottom/RConn1 -- R206/RConn1 -- C106/RConn1 -- Gto6/RConn1
  SaturableReactor/LConn1 -- top/RConn1
  C101/LConn1 -- R101/RConn1
  C102/LConn1 -- R102/RConn1
  R103/RConn1 -- C103/LConn1
  R104/RConn1 -- C104/LConn1
  R105/RConn1 -- C105/LConn1
  R106/RConn1 -- C106/LConn1

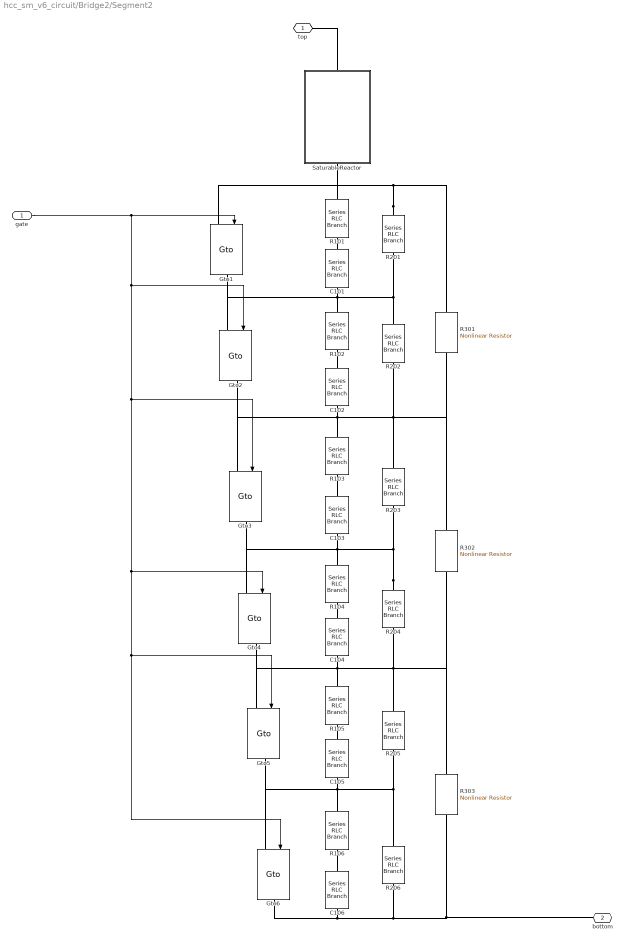
== system hcc_sm_v6_circuit/Bridge2/Segment2 ==
  gate : Inport
  C{101..106} (6 alike) : spsSeriesRLCBranchLib/Series RLC Branch  LConnTagsString=__new0  RConnTagsString=__new0  BranchType=C  Resistance=350  Inductance=107.42e-03  SetiL0=off  InitialCurrent=0  Capacitance=2.2*1e-6  Setx0=off  InitialVoltage=0  Measurements=None
  Gto{1..6} (6 alike) : spsGtoLib/Gto  Ron=0.226e-6  Lon=0  Vf=1.2  Tf=10e-6  Tt=20e-6  IC=0  Rs=161.25e3  Cs=0  Measurements=off
  R{101..106} (6 alike) : spsSeriesRLCBranchLib/Series RLC Branch  LConnTagsString=__new0  RConnTagsString=__new0  BranchType=R  Resistance=36  Inductance=107.42e-03  SetiL0=off  InitialCurrent=0  Capacitance=2.62e-06  Setx0=off  InitialVoltage=0  Measurements=None
  R{201..206} (6 alike) : spsSeriesRLCBranchLib/Series RLC Branch  LConnTagsString=__new0  RConnTagsString=__new0  BranchType=R  Resistance=88  Inductance=107.42e-03  SetiL0=off  InitialCurrent=0  Capacitance=2.62e-06  Setx0=off  InitialVoltage=0  Measurements=None
  R301 : spsNonlinearResistorLib/Nonlinear Resistor  SrcType=Current source  VI=[4400 0.001;5199.92 10;5449.84 100;5700.2 250;5849.8 500;5925.04 750;5999.84 1000;6199.64 2000;6274.84 2500;6325 3000;6600 5500]
  R302 : spsNonlinearResistorLib/Nonlinear Resistor  SrcType=Current source  VI=[4400 0.001;5199.92 10;5449.84 100;5700.2 250;5849.8 500;5925.04 750;5999.84 1000;6199.64 2000;6274.84 2500;6325 3000;6600 5500]
  R303 : spsNonlinearResistorLib/Nonlinear Resistor  SrcType=Current source  VI=[4400 0.001;5199.92 10;5449.84 100;5700.2 250;5849.8 500;5925.04 750;5999.84 1000;6199.64 2000;6274.84 2500;6325 3000;6600 5500]
  SaturableReactor : Subsystem
  top : PMIOPort  Side=Left
  bottom : PMIOPort  Port=2  Side=Right
  wires:
  gate/1 -> Gto3/1, Gto4/1, Gto6/1, Gto5/1, Gto2/1, Gto1/1
  connections:
  R201/RConn1 -- Gto2/LConn1 -- Gto1/RConn1 -- C101/RConn1 -- R102/LConn1 -- R202/LConn1
  R204/LConn1 -- R203/RConn1 -- C103/RConn1 -- Gto4/LConn1 -- Gto3/RConn1 -- R104/LConn1
  R201/LConn1 -- R301/LConn1 -- Gto1/LConn1 -- SaturableReactor/RConn1 -- R101/LConn1
  R205/RConn1 -- C105/RConn1 -- R106/LConn1 -- Gto6/LConn1 -- Gto5/RConn1 -- R206/LConn1
  R202/RConn1 -- R203/LConn1 -- R302/LConn1 -- R301/RConn1 -- C102/RConn1 -- Gto3/LConn1 -- Gto2/RConn1 -- R103/LConn1
  R105/LConn1 -- C104/RConn1 -- Gto5/LConn1 -- Gto4/RConn1 -- R205/LConn1 -- R303/LConn1 -- R302/RConn1 -- R204/RConn1
  R303/RConn1 -- bottom/RConn1 -- R206/RConn1 -- C106/RConn1 -- Gto6/RConn1
  SaturableReactor/LConn1 -- top/RConn1
  C101/LConn1 -- R101/RConn1
  C102/LConn1 -- R102/RConn1
  R103/RConn1 -- C103/LConn1
  R104/RConn1 -- C104/LConn1
  R105/RConn1 -- C105/LConn1
  R106/RConn1 -- C106/LConn1

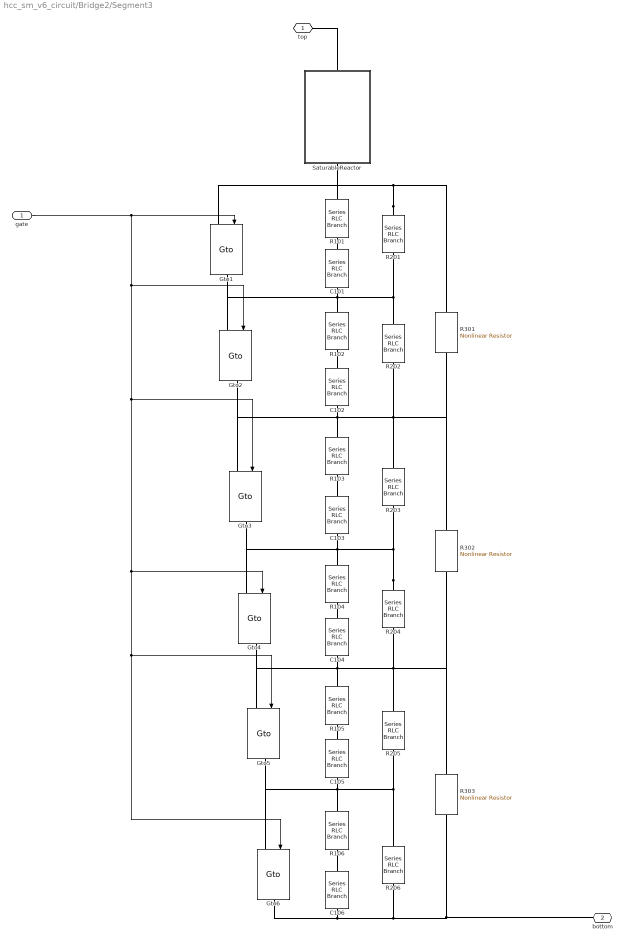
== system hcc_sm_v6_circuit/Bridge2/Segment3 ==
  gate : Inport
  C{101..106} (6 alike) : spsSeriesRLCBranchLib/Series RLC Branch  LConnTagsString=__new0  RConnTagsString=__new0  BranchType=C  Resistance=350  Inductance=107.42e-03  SetiL0=off  InitialCurrent=0  Capacitance=2.2*1e-6  Setx0=off  InitialVoltage=0  Measurements=None
  Gto{1..6} (6 alike) : spsGtoLib/Gto  Ron=0.226e-6  Lon=0  Vf=1.2  Tf=10e-6  Tt=20e-6  IC=0  Rs=161.25e3  Cs=0  Measurements=off
  R{101..106} (6 alike) : spsSeriesRLCBranchLib/Series RLC Branch  LConnTagsString=__new0  RConnTagsString=__new0  BranchType=R  Resistance=36  Inductance=107.42e-03  SetiL0=off  InitialCurrent=0  Capacitance=2.62e-06  Setx0=off  InitialVoltage=0  Measurements=None
  R{201..206} (6 alike) : spsSeriesRLCBranchLib/Series RLC Branch  LConnTagsString=__new0  RConnTagsString=__new0  BranchType=R  Resistance=88  Inductance=107.42e-03  SetiL0=off  InitialCurrent=0  Capacitance=2.62e-06  Setx0=off  InitialVoltage=0  Measurements=None
  R301 : spsNonlinearResistorLib/Nonlinear Resistor  SrcType=Current source  VI=[4400 0.001;5199.92 10;5449.84 100;5700.2 250;5849.8 500;5925.04 750;5999.84 1000;6199.64 2000;6274.84 2500;6325 3000;6600 5500]
  R302 : spsNonlinearResistorLib/Nonlinear Resistor  SrcType=Current source  VI=[4400 0.001;5199.92 10;5449.84 100;5700.2 250;5849.8 500;5925.04 750;5999.84 1000;6199.64 2000;6274.84 2500;6325 3000;6600 5500]
  R303 : spsNonlinearResistorLib/Nonlinear Resistor  SrcType=Current source  VI=[4400 0.001;5199.92 10;5449.84 100;5700.2 250;5849.8 500;5925.04 750;5999.84 1000;6199.64 2000;6274.84 2500;6325 3000;6600 5500]
  SaturableReactor : Subsystem
  top : PMIOPort  Side=Left
  bottom : PMIOPort  Port=2  Side=Right
  wires:
  gate/1 -> Gto3/1, Gto4/1, Gto6/1, Gto5/1, Gto2/1, Gto1/1
  connections:
  R201/RConn1 -- Gto2/LConn1 -- Gto1/RConn1 -- C101/RConn1 -- R102/LConn1 -- R202/LConn1
  R204/LConn1 -- R203/RConn1 -- C103/RConn1 -- Gto4/LConn1 -- Gto3/RConn1 -- R104/LConn1
  R201/LConn1 -- R301/LConn1 -- Gto1/LConn1 -- SaturableReactor/RConn1 -- R101/LConn1
  R205/RConn1 -- C105/RConn1 -- R106/LConn1 -- Gto6/LConn1 -- Gto5/RConn1 -- R206/LConn1
  R202/RConn1 -- R203/LConn1 -- R302/LConn1 -- R301/RConn1 -- C102/RConn1 -- Gto3/LConn1 -- Gto2/RConn1 -- R103/LConn1
  R105/LConn1 -- C104/RConn1 -- Gto5/LConn1 -- Gto4/RConn1 -- R205/LConn1 -- R303/LConn1 -- R302/RConn1 -- R204/RConn1
  R303/RConn1 -- bottom/RConn1 -- R206/RConn1 -- C106/RConn1 -- Gto6/RConn1
  SaturableReactor/LConn1 -- top/RConn1
  C101/LConn1 -- R101/RConn1
  C102/LConn1 -- R102/RConn1
  R103/RConn1 -- C103/LConn1
  R104/RConn1 -- C104/LConn1
  R105/RConn1 -- C105/LConn1
  R106/RConn1 -- C106/LConn1

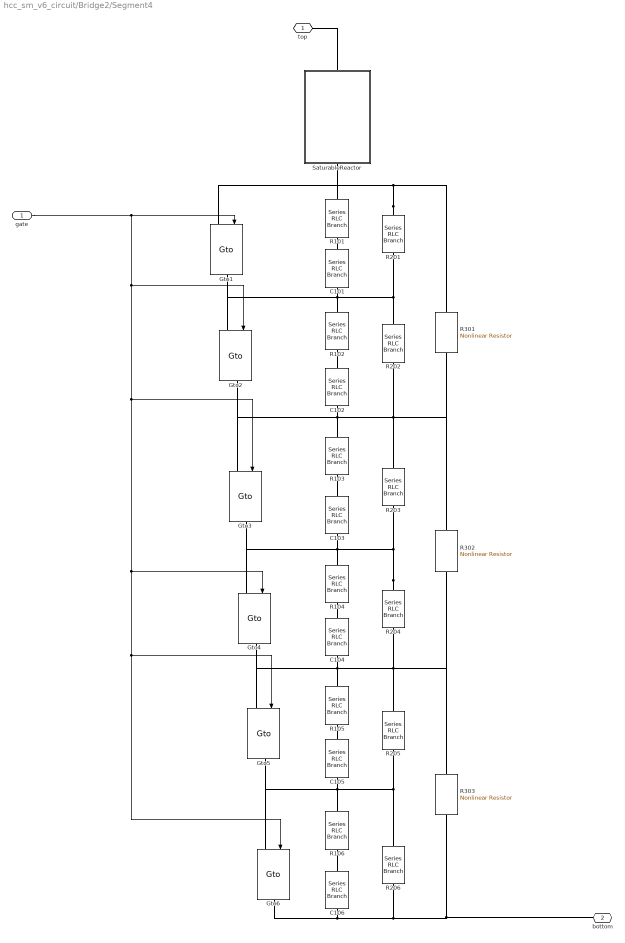
== system hcc_sm_v6_circuit/Bridge2/Segment4 ==
  gate : Inport
  C{101..106} (6 alike) : spsSeriesRLCBranchLib/Series RLC Branch  LConnTagsString=__new0  RConnTagsString=__new0  BranchType=C  Resistance=350  Inductance=107.42e-03  SetiL0=off  InitialCurrent=0  Capacitance=2.2*1e-6  Setx0=off  InitialVoltage=0  Measurements=None
  Gto{1..6} (6 alike) : spsGtoLib/Gto  Ron=0.226e-6  Lon=0  Vf=1.2  Tf=10e-6  Tt=20e-6  IC=0  Rs=161.25e3  Cs=0  Measurements=off
  R{101..106} (6 alike) : spsSeriesRLCBranchLib/Series RLC Branch  LConnTagsString=__new0  RConnTagsString=__new0  BranchType=R  Resistance=36  Inductance=107.42e-03  SetiL0=off  InitialCurrent=0  Capacitance=2.62e-06  Setx0=off  InitialVoltage=0  Measurements=None
  R{201..206} (6 alike) : spsSeriesRLCBranchLib/Series RLC Branch  LConnTagsString=__new0  RConnTagsString=__new0  BranchType=R  Resistance=88  Inductance=107.42e-03  SetiL0=off  InitialCurrent=0  Capacitance=2.62e-06  Setx0=off  InitialVoltage=0  Measurements=None
  R301 : spsNonlinearResistorLib/Nonlinear Resistor  SrcType=Current source  VI=[4400 0.001;5199.92 10;5449.84 100;5700.2 250;5849.8 500;5925.04 750;5999.84 1000;6199.64 2000;6274.84 2500;6325 3000;6600 5500]
  R302 : spsNonlinearResistorLib/Nonlinear Resistor  SrcType=Current source  VI=[4400 0.001;5199.92 10;5449.84 100;5700.2 250;5849.8 500;5925.04 750;5999.84 1000;6199.64 2000;6274.84 2500;6325 3000;6600 5500]
  R303 : spsNonlinearResistorLib/Nonlinear Resistor  SrcType=Current source  VI=[4400 0.001;5199.92 10;5449.84 100;5700.2 250;5849.8 500;5925.04 750;5999.84 1000;6199.64 2000;6274.84 2500;6325 3000;6600 5500]
  SaturableReactor : Subsystem
  top : PMIOPort  Side=Left
  bottom : PMIOPort  Port=2  Side=Right
  wires:
  gate/1 -> Gto3/1, Gto4/1, Gto6/1, Gto5/1, Gto2/1, Gto1/1
  connections:
  R201/RConn1 -- Gto2/LConn1 -- Gto1/RConn1 -- C101/RConn1 -- R102/LConn1 -- R202/LConn1
  R204/LConn1 -- R203/RConn1 -- C103/RConn1 -- Gto4/LConn1 -- Gto3/RConn1 -- R104/LConn1
  R201/LConn1 -- R301/LConn1 -- Gto1/LConn1 -- SaturableReactor/RConn1 -- R101/LConn1
  R205/RConn1 -- C105/RConn1 -- R106/LConn1 -- Gto6/LConn1 -- Gto5/RConn1 -- R206/LConn1
  R202/RConn1 -- R203/LConn1 -- R302/LConn1 -- R301/RConn1 -- C102/RConn1 -- Gto3/LConn1 -- Gto2/RConn1 -- R103/LConn1
  R105/LConn1 -- C104/RConn1 -- Gto5/LConn1 -- Gto4/RConn1 -- R205/LConn1 -- R303/LConn1 -- R302/RConn1 -- R204/RConn1
  R303/RConn1 -- bottom/RConn1 -- R206/RConn1 -- C106/RConn1 -- Gto6/RConn1
  SaturableReactor/LConn1 -- top/RConn1
  C101/LConn1 -- R101/RConn1
  C102/LConn1 -- R102/RConn1
  R103/RConn1 -- C103/LConn1
  R104/RConn1 -- C104/LConn1
  R105/RConn1 -- C105/LConn1
  R106/RConn1 -- C106/LConn1

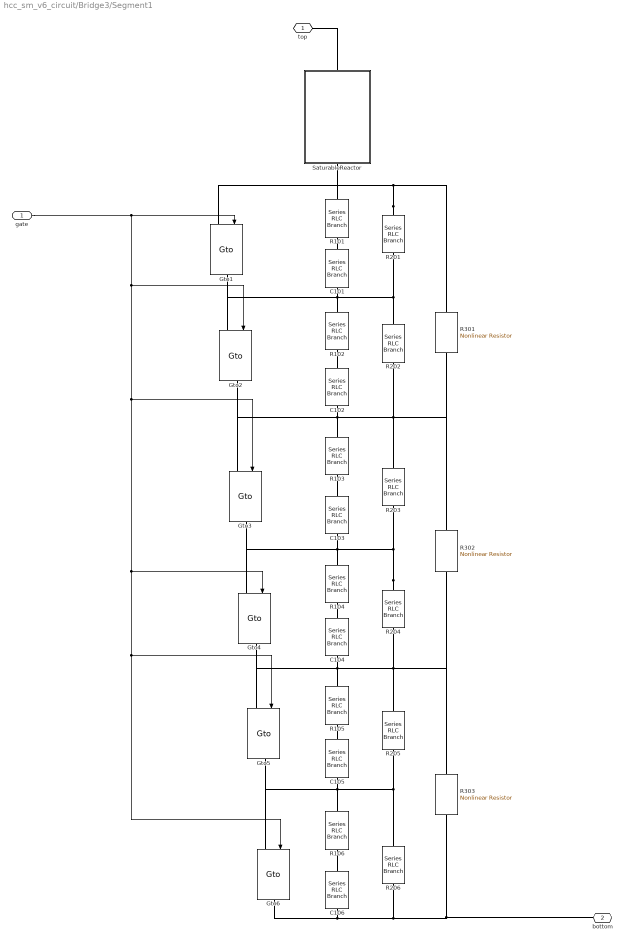
== system hcc_sm_v6_circuit/Bridge3/Segment1 ==
  gate : Inport
  C{101..106} (6 alike) : spsSeriesRLCBranchLib/Series RLC Branch  LConnTagsString=__new0  RConnTagsString=__new0  BranchType=C  Resistance=350  Inductance=107.42e-03  SetiL0=off  InitialCurrent=0  Capacitance=2.2*1e-6  Setx0=off  InitialVoltage=0  Measurements=None
  Gto{1..6} (6 alike) : spsGtoLib/Gto  Ron=0.226e-6  Lon=0  Vf=1.2  Tf=10e-6  Tt=20e-6  IC=0  Rs=161.25e3  Cs=0  Measurements=off
  R{101..106} (6 alike) : spsSeriesRLCBranchLib/Series RLC Branch  LConnTagsString=__new0  RConnTagsString=__new0  BranchType=R  Resistance=36  Inductance=107.42e-03  SetiL0=off  InitialCurrent=0  Capacitance=2.62e-06  Setx0=off  InitialVoltage=0  Measurements=None
  R{201..206} (6 alike) : spsSeriesRLCBranchLib/Series RLC Branch  LConnTagsString=__new0  RConnTagsString=__new0  BranchType=R  Resistance=88  Inductance=107.42e-03  SetiL0=off  InitialCurrent=0  Capacitance=2.62e-06  Setx0=off  InitialVoltage=0  Measurements=None
  R301 : spsNonlinearResistorLib/Nonlinear Resistor  SrcType=Current source  VI=[4400 0.001;5199.92 10;5449.84 100;5700.2 250;5849.8 500;5925.04 750;5999.84 1000;6199.64 2000;6274.84 2500;6325 3000;6600 5500]
  R302 : spsNonlinearResistorLib/Nonlinear Resistor  SrcType=Current source  VI=[4400 0.001;5199.92 10;5449.84 100;5700.2 250;5849.8 500;5925.04 750;5999.84 1000;6199.64 2000;6274.84 2500;6325 3000;6600 5500]
  R303 : spsNonlinearResistorLib/Nonlinear Resistor  SrcType=Current source  VI=[4400 0.001;5199.92 10;5449.84 100;5700.2 250;5849.8 500;5925.04 750;5999.84 1000;6199.64 2000;6274.84 2500;6325 3000;6600 5500]
  SaturableReactor : Subsystem
  top : PMIOPort  Side=Left
  bottom : PMIOPort  Port=2  Side=Right
  wires:
  gate/1 -> Gto3/1, Gto4/1, Gto6/1, Gto5/1, Gto2/1, Gto1/1
  connections:
  R201/RConn1 -- Gto2/LConn1 -- Gto1/RConn1 -- C101/RConn1 -- R102/LConn1 -- R202/LConn1
  R204/LConn1 -- R203/RConn1 -- C103/RConn1 -- Gto4/LConn1 -- Gto3/RConn1 -- R104/LConn1
  R201/LConn1 -- R301/LConn1 -- Gto1/LConn1 -- SaturableReactor/RConn1 -- R101/LConn1
  R205/RConn1 -- C105/RConn1 -- R106/LConn1 -- Gto6/LConn1 -- Gto5/RConn1 -- R206/LConn1
  R202/RConn1 -- R203/LConn1 -- R302/LConn1 -- R301/RConn1 -- C102/RConn1 -- Gto3/LConn1 -- Gto2/RConn1 -- R103/LConn1
  R105/LConn1 -- C104/RConn1 -- Gto5/LConn1 -- Gto4/RConn1 -- R205/LConn1 -- R303/LConn1 -- R302/RConn1 -- R204/RConn1
  R303/RConn1 -- bottom/RConn1 -- R206/RConn1 -- C106/RConn1 -- Gto6/RConn1
  SaturableReactor/LConn1 -- top/RConn1
  C101/LConn1 -- R101/RConn1
  C102/LConn1 -- R102/RConn1
  R103/RConn1 -- C103/LConn1
  R104/RConn1 -- C104/LConn1
  R105/RConn1 -- C105/LConn1
  R106/RConn1 -- C106/LConn1

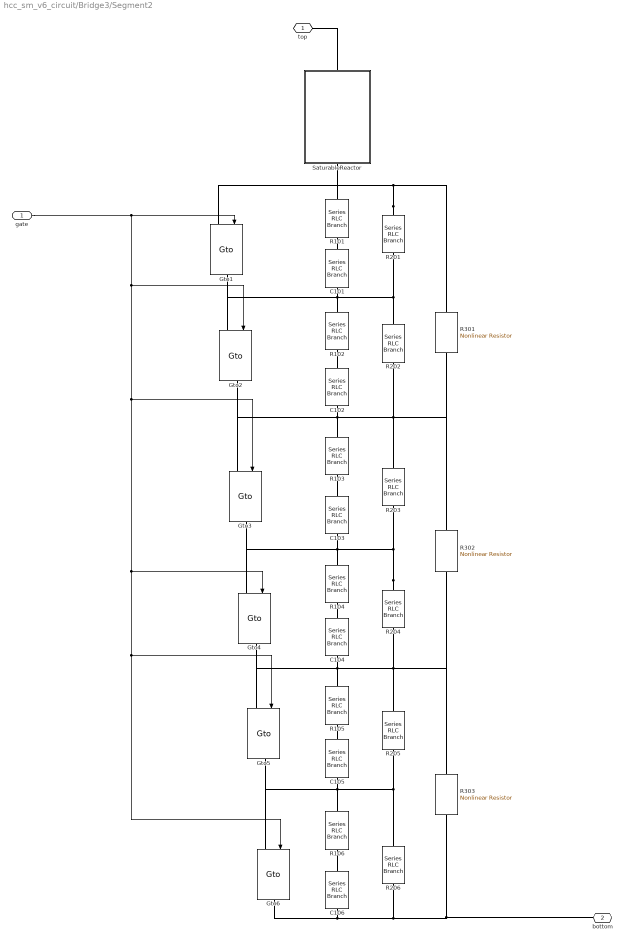
== system hcc_sm_v6_circuit/Bridge3/Segment2 ==
  gate : Inport
  C{101..106} (6 alike) : spsSeriesRLCBranchLib/Series RLC Branch  LConnTagsString=__new0  RConnTagsString=__new0  BranchType=C  Resistance=350  Inductance=107.42e-03  SetiL0=off  InitialCurrent=0  Capacitance=2.2*1e-6  Setx0=off  InitialVoltage=0  Measurements=None
  Gto{1..6} (6 alike) : spsGtoLib/Gto  Ron=0.226e-6  Lon=0  Vf=1.2  Tf=10e-6  Tt=20e-6  IC=0  Rs=161.25e3  Cs=0  Measurements=off
  R{101..106} (6 alike) : spsSeriesRLCBranchLib/Series RLC Branch  LConnTagsString=__new0  RConnTagsString=__new0  BranchType=R  Resistance=36  Inductance=107.42e-03  SetiL0=off  InitialCurrent=0  Capacitance=2.62e-06  Setx0=off  InitialVoltage=0  Measurements=None
  R{201..206} (6 alike) : spsSeriesRLCBranchLib/Series RLC Branch  LConnTagsString=__new0  RConnTagsString=__new0  BranchType=R  Resistance=88  Inductance=107.42e-03  SetiL0=off  InitialCurrent=0  Capacitance=2.62e-06  Setx0=off  InitialVoltage=0  Measurements=None
  R301 : spsNonlinearResistorLib/Nonlinear Resistor  SrcType=Current source  VI=[4400 0.001;5199.92 10;5449.84 100;5700.2 250;5849.8 500;5925.04 750;5999.84 1000;6199.64 2000;6274.84 2500;6325 3000;6600 5500]
  R302 : spsNonlinearResistorLib/Nonlinear Resistor  SrcType=Current source  VI=[4400 0.001;5199.92 10;5449.84 100;5700.2 250;5849.8 500;5925.04 750;5999.84 1000;6199.64 2000;6274.84 2500;6325 3000;6600 5500]
  R303 : spsNonlinearResistorLib/Nonlinear Resistor  SrcType=Current source  VI=[4400 0.001;5199.92 10;5449.84 100;5700.2 250;5849.8 500;5925.04 750;5999.84 1000;6199.64 2000;6274.84 2500;6325 3000;6600 5500]
  SaturableReactor : Subsystem
  top : PMIOPort  Side=Left
  bottom : PMIOPort  Port=2  Side=Right
  wires:
  gate/1 -> Gto3/1, Gto4/1, Gto6/1, Gto5/1, Gto2/1, Gto1/1
  connections:
  R201/RConn1 -- Gto2/LConn1 -- Gto1/RConn1 -- C101/RConn1 -- R102/LConn1 -- R202/LConn1
  R204/LConn1 -- R203/RConn1 -- C103/RConn1 -- Gto4/LConn1 -- Gto3/RConn1 -- R104/LConn1
  R201/LConn1 -- R301/LConn1 -- Gto1/LConn1 -- SaturableReactor/RConn1 -- R101/LConn1
  R205/RConn1 -- C105/RConn1 -- R106/LConn1 -- Gto6/LConn1 -- Gto5/RConn1 -- R206/LConn1
  R202/RConn1 -- R203/LConn1 -- R302/LConn1 -- R301/RConn1 -- C102/RConn1 -- Gto3/LConn1 -- Gto2/RConn1 -- R103/LConn1
  R105/LConn1 -- C104/RConn1 -- Gto5/LConn1 -- Gto4/RConn1 -- R205/LConn1 -- R303/LConn1 -- R302/RConn1 -- R204/RConn1
  R303/RConn1 -- bottom/RConn1 -- R206/RConn1 -- C106/RConn1 -- Gto6/RConn1
  SaturableReactor/LConn1 -- top/RConn1
  C101/LConn1 -- R101/RConn1
  C102/LConn1 -- R102/RConn1
  R103/RConn1 -- C103/LConn1
  R104/RConn1 -- C104/LConn1
  R105/RConn1 -- C105/LConn1
  R106/RConn1 -- C106/LConn1

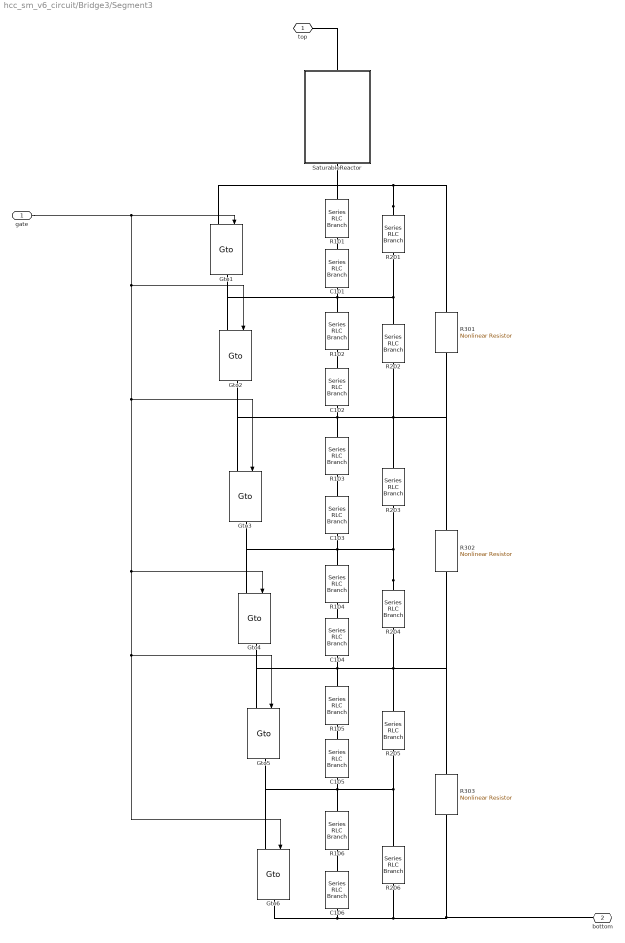
== system hcc_sm_v6_circuit/Bridge3/Segment3 ==
  gate : Inport
  C{101..106} (6 alike) : spsSeriesRLCBranchLib/Series RLC Branch  LConnTagsString=__new0  RConnTagsString=__new0  BranchType=C  Resistance=350  Inductance=107.42e-03  SetiL0=off  InitialCurrent=0  Capacitance=2.2*1e-6  Setx0=off  InitialVoltage=0  Measurements=None
  Gto{1..6} (6 alike) : spsGtoLib/Gto  Ron=0.226e-6  Lon=0  Vf=1.2  Tf=10e-6  Tt=20e-6  IC=0  Rs=161.25e3  Cs=0  Measurements=off
  R{101..106} (6 alike) : spsSeriesRLCBranchLib/Series RLC Branch  LConnTagsString=__new0  RConnTagsString=__new0  BranchType=R  Resistance=36  Inductance=107.42e-03  SetiL0=off  InitialCurrent=0  Capacitance=2.62e-06  Setx0=off  InitialVoltage=0  Measurements=None
  R{201..206} (6 alike) : spsSeriesRLCBranchLib/Series RLC Branch  LConnTagsString=__new0  RConnTagsString=__new0  BranchType=R  Resistance=88  Inductance=107.42e-03  SetiL0=off  InitialCurrent=0  Capacitance=2.62e-06  Setx0=off  InitialVoltage=0  Measurements=None
  R301 : spsNonlinearResistorLib/Nonlinear Resistor  SrcType=Current source  VI=[4400 0.001;5199.92 10;5449.84 100;5700.2 250;5849.8 500;5925.04 750;5999.84 1000;6199.64 2000;6274.84 2500;6325 3000;6600 5500]
  R302 : spsNonlinearResistorLib/Nonlinear Resistor  SrcType=Current source  VI=[4400 0.001;5199.92 10;5449.84 100;5700.2 250;5849.8 500;5925.04 750;5999.84 1000;6199.64 2000;6274.84 2500;6325 3000;6600 5500]
  R303 : spsNonlinearResistorLib/Nonlinear Resistor  SrcType=Current source  VI=[4400 0.001;5199.92 10;5449.84 100;5700.2 250;5849.8 500;5925.04 750;5999.84 1000;6199.64 2000;6274.84 2500;6325 3000;6600 5500]
  SaturableReactor : Subsystem
  top : PMIOPort  Side=Left
  bottom : PMIOPort  Port=2  Side=Right
  wires:
  gate/1 -> Gto3/1, Gto4/1, Gto6/1, Gto5/1, Gto2/1, Gto1/1
  connections:
  R201/RConn1 -- Gto2/LConn1 -- Gto1/RConn1 -- C101/RConn1 -- R102/LConn1 -- R202/LConn1
  R204/LConn1 -- R203/RConn1 -- C103/RConn1 -- Gto4/LConn1 -- Gto3/RConn1 -- R104/LConn1
  R201/LConn1 -- R301/LConn1 -- Gto1/LConn1 -- SaturableReactor/RConn1 -- R101/LConn1
  R205/RConn1 -- C105/RConn1 -- R106/LConn1 -- Gto6/LConn1 -- Gto5/RConn1 -- R206/LConn1
  R202/RConn1 -- R203/LConn1 -- R302/LConn1 -- R301/RConn1 -- C102/RConn1 -- Gto3/LConn1 -- Gto2/RConn1 -- R103/LConn1
  R105/LConn1 -- C104/RConn1 -- Gto5/LConn1 -- Gto4/RConn1 -- R205/LConn1 -- R303/LConn1 -- R302/RConn1 -- R204/RConn1
  R303/RConn1 -- bottom/RConn1 -- R206/RConn1 -- C106/RConn1 -- Gto6/RConn1
  SaturableReactor/LConn1 -- top/RConn1
  C101/LConn1 -- R101/RConn1
  C102/LConn1 -- R102/RConn1
  R103/RConn1 -- C103/LConn1
  R104/RConn1 -- C104/LConn1
  R105/RConn1 -- C105/LConn1
  R106/RConn1 -- C106/LConn1

== system hcc_sm_v6_circuit/Bridge3/Segment4 ==
  gate : Inport
  C{101..106} (6 alike) : spsSeriesRLCBranchLib/Series RLC Branch  LConnTagsString=__new0  RConnTagsString=__new0  BranchType=C  Resistance=350  Inductance=107.42e-03  SetiL0=off  InitialCurrent=0  Capacitance=2.2*1e-6  Setx0=off  InitialVoltage=0  Measurements=None
  Gto{1..6} (6 alike) : spsGtoLib/Gto  Ron=0.226e-6  Lon=0  Vf=1.2  Tf=10e-6  Tt=20e-6  IC=0  Rs=161.25e3  Cs=0  Measurements=off
  R{101..106} (6 alike) : spsSeriesRLCBranchLib/Series RLC Branch  LConnTagsString=__new0  RConnTagsString=__new0  BranchType=R  Resistance=36  Inductance=107.42e-03  SetiL0=off  InitialCurrent=0  Capacitance=2.62e-06  Setx0=off  InitialVoltage=0  Measurements=None
  R{201..206} (6 alike) : spsSeriesRLCBranchLib/Series RLC Branch  LConnTagsString=__new0  RConnTagsString=__new0  BranchType=R  Resistance=88  Inductance=107.42e-03  SetiL0=off  InitialCurrent=0  Capacitance=2.62e-06  Setx0=off  InitialVoltage=0  Measurements=None
  R301 : spsNonlinearResistorLib/Nonlinear Resistor  SrcType=Current source  VI=[4400 0.001;5199.92 10;5449.84 100;5700.2 250;5849.8 500;5925.04 750;5999.84 1000;6199.64 2000;6274.84 2500;6325 3000;6600 5500]
  R302 : spsNonlinearResistorLib/Nonlinear Resistor  SrcType=Current source  VI=[4400 0.001;5199.92 10;5449.84 100;5700.2 250;5849.8 500;5925.04 750;5999.84 1000;6199.64 2000;6274.84 2500;6325 3000;6600 5500]
  R303 : spsNonlinearResistorLib/Nonlinear Resistor  SrcType=Current source  VI=[4400 0.001;5199.92 10;5449.84 100;5700.2 250;5849.8 500;5925.04 750;5999.84 1000;6199.64 2000;6274.84 2500;6325 3000;6600 5500]
  SaturableReactor : Subsystem
  top : PMIOPort  Side=Left
  bottom : PMIOPort  Port=2  Side=Right
  wires:
  gate/1 -> Gto3/1, Gto4/1, Gto6/1, Gto5/1, Gto2/1, Gto1/1
  connections:
  R201/RConn1 -- Gto2/LConn1 -- Gto1/RConn1 -- C101/RConn1 -- R102/LConn1 -- R202/LConn1
  R204/LConn1 -- R203/RConn1 -- C103/RConn1 -- Gto4/LConn1 -- Gto3/RConn1 -- R104/LConn1
  R201/LConn1 -- R301/LConn1 -- Gto1/LConn1 -- SaturableReactor/RConn1 -- R101/LConn1
  R205/RConn1 -- C105/RConn1 -- R106/LConn1 -- Gto6/LConn1 -- Gto5/RConn1 -- R206/LConn1
  R202/RConn1 -- R203/LConn1 -- R302/LConn1 -- R301/RConn1 -- C102/RConn1 -- Gto3/LConn1 -- Gto2/RConn1 -- R103/LConn1
  R105/LConn1 -- C104/RConn1 -- Gto5/LConn1 -- Gto4/RConn1 -- R205/LConn1 -- R303/LConn1 -- R302/RConn1 -- R204/RConn1
  R303/RConn1 -- bottom/RConn1 -- R206/RConn1 -- C106/RConn1 -- Gto6/RConn1
  SaturableReactor/LConn1 -- top/RConn1
  C101/LConn1 -- R101/RConn1
  C102/LConn1 -- R102/RConn1
  R103/RConn1 -- C103/LConn1
  R104/RConn1 -- C104/LConn1
  R105/RConn1 -- C105/LConn1
  R106/RConn1 -- C106/LConn1

== system hcc_sm_v6_circuit/Bridge4/Segment1 ==
  gate : Inport
  C{101..106} (6 alike) : spsSeriesRLCBranchLib/Series RLC Branch  LConnTagsString=__new0  RConnTagsString=__new0  BranchType=C  Resistance=350  Inductance=107.42e-03  SetiL0=off  InitialCurrent=0  Capacitance=2.2*1e-6  Setx0=off  InitialVoltage=0  Measurements=None
  Gto{1..6} (6 alike) : spsGtoLib/Gto  Ron=0.226e-6  Lon=0  Vf=1.2  Tf=10e-6  Tt=20e-6  IC=0  Rs=161.25e3  Cs=0  Measurements=off
  R{101..106} (6 alike) : spsSeriesRLCBranchLib/Series RLC Branch  LConnTagsString=__new0  RConnTagsString=__new0  BranchType=R  Resistance=36  Inductance=107.42e-03  SetiL0=off  InitialCurrent=0  Capacitance=2.62e-06  Setx0=off  InitialVoltage=0  Measurements=None
  R{201..206} (6 alike) : spsSeriesRLCBranchLib/Series RLC Branch  LConnTagsString=__new0  RConnTagsString=__new0  BranchType=R  Resistance=88  Inductance=107.42e-03  SetiL0=off  InitialCurrent=0  Capacitance=2.62e-06  Setx0=off  InitialVoltage=0  Measurements=None
  R301 : spsNonlinearResistorLib/Nonlinear Resistor  SrcType=Current source  VI=[4400 0.001;5199.92 10;5449.84 100;5700.2 250;5849.8 500;5925.04 750;5999.84 1000;6199.64 2000;6274.84 2500;6325 3000;6600 5500]
  R302 : spsNonlinearResistorLib/Nonlinear Resistor  SrcType=Current source  VI=[4400 0.001;5199.92 10;5449.84 100;5700.2 250;5849.8 500;5925.04 750;5999.84 1000;6199.64 2000;6274.84 2500;6325 3000;6600 5500]
  R303 : spsNonlinearResistorLib/Nonlinear Resistor  SrcType=Current source  VI=[4400 0.001;5199.92 10;5449.84 100;5700.2 250;5849.8 500;5925.04 750;5999.84 1000;6199.64 2000;6274.84 2500;6325 3000;6600 5500]
  SaturableReactor : Subsystem
  top : PMIOPort  Side=Left
  bottom : PMIOPort  Port=2  Side=Right
  wires:
  gate/1 -> Gto3/1, Gto4/1, Gto6/1, Gto5/1, Gto2/1, Gto1/1
  connections:
  R201/RConn1 -- Gto2/LConn1 -- Gto1/RConn1 -- C101/RConn1 -- R102/LConn1 -- R202/LConn1
  R204/LConn1 -- R203/RConn1 -- C103/RConn1 -- Gto4/LConn1 -- Gto3/RConn1 -- R104/LConn1
  R201/LConn1 -- R301/LConn1 -- Gto1/LConn1 -- SaturableReactor/RConn1 -- R101/LConn1
  R205/RConn1 -- C105/RConn1 -- R106/LConn1 -- Gto6/LConn1 -- Gto5/RConn1 -- R206/LConn1
  R202/RConn1 -- R203/LConn1 -- R302/LConn1 -- R301/RConn1 -- C102/RConn1 -- Gto3/LConn1 -- Gto2/RConn1 -- R103/LConn1
  R105/LConn1 -- C104/RConn1 -- Gto5/LConn1 -- Gto4/RConn1 -- R205/LConn1 -- R303/LConn1 -- R302/RConn1 -- R204/RConn1
  R303/RConn1 -- bottom/RConn1 -- R206/RConn1 -- C106/RConn1 -- Gto6/RConn1
  SaturableReactor/LConn1 -- top/RConn1
  C101/LConn1 -- R101/RConn1
  C102/LConn1 -- R102/RConn1
  R103/RConn1 -- C103/LConn1
  R104/RConn1 -- C104/LConn1
  R105/RConn1 -- C105/LConn1
  R106/RConn1 -- C106/LConn1
